simulink model "dt_crff3_non_ideal"  (R2025b)
settings: Solver=VariableStepAuto  StartTime=0.0  StopTime=10.0  RelTol=1e-3
model workspace (MAT data in the model file):
  Delay_1 = [0 0 0]
  ENOB_1 = 3.82010676042
  FUNDF_1 = [99.7346662356 299.517854363]
  FUNDX_1 = [15.4853229373 -15.5048641556]
  IMODF_1 = [nan 499.461934629]
  IMODX_1 = [nan -22.9176650349]
  NoiseFloor_1 = -39.8464180971
  OIP3_1 = nan
  SFDR_1 = 30.038334306
  SINAD_1 = 24.7570426978
  SNR_1 = 26.1601373132
  THD_1 = -30.1916968059
  delay_1 = [0 0 0]
undefined symbols (not defined in the file): DiscIntNeverNeededParam, Fs
libraries: dspmlti4 x5, msbAdcMeasurements x1, cstblocks x1, dspobslib x1, simulink x1
settings Model: Creator=divya  LastModifiedBy=divya

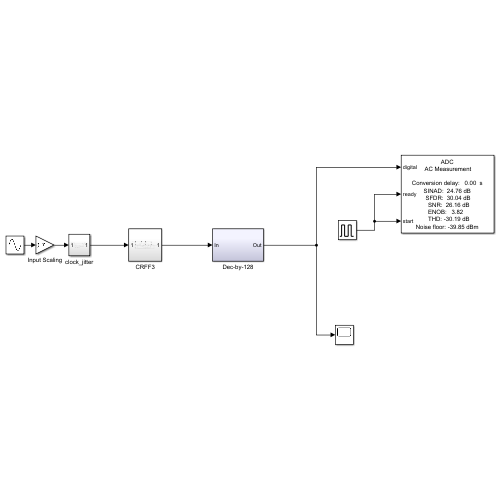
[thumbnail: Simulink's stored preview of the top-level diagram]
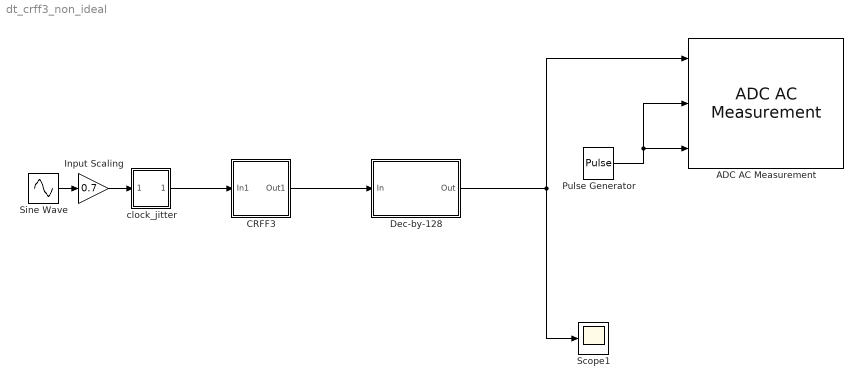
== system dt_crff3_non_ideal ==
  ADC AC Measurement : msbAdcMeasurements/ADC AC Measurement  DistortionMeasurement=Harmonic  InputFrequency=100  Method=Filter bank (slower, requires extra simulation time)  RBW=0.97656  AutoSetRBW=on  NBits=18  Frequency=512e3/512  HoldOffTime=0  OutputToWorkspace=on  VariableName=adc_ac_out  ShowSpectrum=off
      link override ADC AC Measurement/ADC AC Measurement Spectrum Analyzer: YLimits=[-137.7231 -38.3847]
  CRFF3 : Subsystem
  Dec-by-128 : Subsystem  Tag=BlockMethodSubSystem
  Input Scaling : Gain  Gain=0.7
  Pulse Generator : DiscretePulseGenerator  PulseType=Time based  Period=1/1e3  PulseWidth=50
  Scope1 : Scope
      settings: ActiveDisplayYMinimum=-0.48077534934995808  ActiveDisplayYMaximum=0.47749694685441174
  Sine Wave : Sin  Amplitude=0.5  Frequency=628  SampleTime=0
  clock_jitter : Subsystem
  wires:
  Sine Wave/1 -> Input Scaling/1
  clock_jitter/1(Out1) -> CRFF3/1(In1)
  Input Scaling/1 -> clock_jitter/1(In1)
  Pulse Generator/1 -> ADC AC Measurement/3, ADC AC Measurement/2
  Dec-by-128/1(Out) -> ADC AC Measurement/1, Scope1/1
  CRFF3/1(Out1) -> Dec-by-128/1(In)

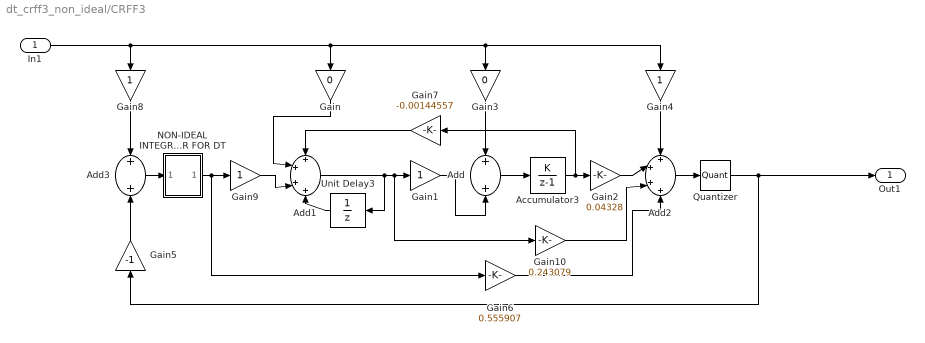
== system dt_crff3_non_ideal/CRFF3 ==
  In1 : Inport
  Accumulator3 : DiscreteIntegrator  RequirementInfo={} %GIDa_84b8a85e_70bd_4012_ac1e_63614c4be6d6  IntegratorMethod=Accumulation: Forward Euler  SampleTime=1/(2e3*256)  ICPrevOutput=DiscIntNeverNeededParam  ICPrevScaledInput=DiscIntNeverNeededParam
  Add : Sum  RequirementInfo={} %GIDa_1bae6441_7ec0_4b3d_934d_76e9e43c9b7e
  Add1 : Sum  RequirementInfo={} %GIDa_a9ab647b_ef6c_44ae_a7d7_07674ff6e1b7  Inputs=++++
  Add2 : Sum  RequirementInfo={} %GIDa_90ab26b4_1233_497e_bd04_95e33db7a632  Inputs=++++
  Add3 : Sum  RequirementInfo={} %GIDa_7332c942_930d_40b4_92c2_cb866450a1ff
  Gain : Gain  RequirementInfo={} %GIDa_66f1e292_dda5_4196_a756_d7da6c9f4ec1  Gain=0
  Gain1 : Gain  RequirementInfo={} %GIDa_65ba529b_3bb8_47a6_991c_193e84d935ec
  Gain10 : Gain  RequirementInfo={} %GIDa_9d9f86ed_3f68_4820_a7bb_2b036d160bea  Gain=0.243079
  Gain2 : Gain  RequirementInfo={} %GIDa_aff9fc4e_08da_4d4c_a30b_0e4ade6494bf  Gain=0.04328
  Gain3 : Gain  RequirementInfo={} %GIDa_9119ba48_5aaa_4b92_8d55_fe7266434502  Gain=0
  Gain4 : Gain  RequirementInfo={} %GIDa_0e2722ef_9053_4d44_905a_33326b2b6931
  Gain5 : Gain  RequirementInfo={} %GIDa_f0a11f36_a50f_4b52_8fee_37920b06259d  Gain=-1
  Gain6 : Gain  RequirementInfo={} %GIDa_c76b328f_db54_4ce8_9437_510e711bab7a  Gain=0.555907
  Gain7 : Gain  RequirementInfo={} %GIDa_74793299_c4f9_4dc2_b47d_1811f6d964e4  Gain=-0.00144557
  Gain8 : Gain  RequirementInfo={} %GIDa_eaa10ee5_6284_4d1e_87e1_14929015d833
  Gain9 : Gain  RequirementInfo={} %GIDa_87574565_9502_45cc_a9fb_7b5e642d0bb9
  NON-IDEAL INTEGRATOR FOR DT : Subsystem
  Quantizer : Quantizer  RequirementInfo={} %GIDa_8abe0c8b_02fb_4844_986b_6a962a179ce5  QuantizationInterval=1
  Unit Delay3 : UnitDelay  SampleTime=1/(2e3*256)  HasFrameUpgradeWarning=on
  Out1 : Outport
  wires:
  Gain6/1 -> Add2/4
  Add1/1 -> Unit Delay3/1, Gain10/1, Gain1/1
  Accumulator3/1 -> Gain7/1, Gain2/1
  NON-IDEAL INTEGRATOR FOR DT/1(Out1) -> Gain9/1, Gain6/1
  Unit Delay3/1 -> Add1/4
  Gain9/1 -> Add1/3
  Gain8/1 -> Add3/1
  In1/1 -> Gain8/1, Gain/1, Gain3/1, Gain4/1
  Gain5/1 -> Add3/2
  Gain2/1 -> Add2/2
  Gain10/1 -> Add2/3
  Gain3/1 -> Add/1
  Gain/1 -> Add1/2
  Add2/1 -> Quantizer/1
  Gain7/1 -> Add1/1
  Quantizer/1 -> Out1/1, Gain5/1
  Gain4/1 -> Add2/1
  Gain1/1 -> Add/2
  Add3/1 -> NON-IDEAL INTEGRATOR FOR DT/1(In2)
  Add/1 -> Accumulator3/1

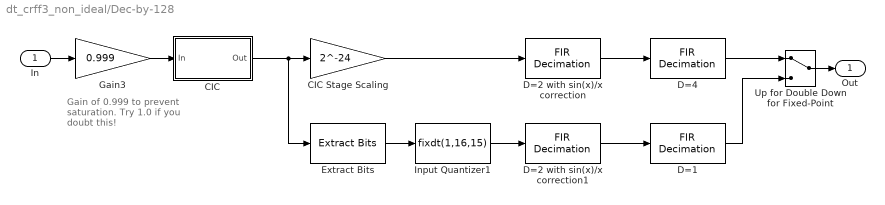
== system dt_crff3_non_ideal/Dec-by-128 ==
  note: Gain of 0.999
      |  to prevent saturation.
      | Try 1.0 if you doubt this!
  In : Inport
  CIC : Subsystem  Tag=BlockMethodSubSystem
  CIC Stage Scaling : Gain  Gain=2^-24  OutDataTypeStr=double
  D=1 : dspmlti4/FIR Decimation  Tag=BlockMethodSubSystem  FilterSource=Dialog parameters  h=[3.91622882568566e-005 6.87965858042108e-005 -4.54214374064863e-005 -0.000494371495641253 -0.00130180300923401 -0.00208967903904167 -0.00212227242054207 -0.000820466891279789 0.00150204580522739 0.00336930831020411 0.00293785704853453 -0.000377156856911545 -0.00470730589029979 -0.00641725180832836 -0.00285434238807273 0.00468881704747952 0.0106481610663031 0.00886595641260817 -0.00177682957707149 -0.0144760924096176 -0.0180887636371107 -0.00603326390232397 0.0159987454589339 0.0309930177585429 0.0221515825094605 -0.011846123967549 -0.04979943488328 -0.0572170491759349 -0.00847489358036981 0.0923226139783473 0.207458472082029 0.283964644704709 0.283964644704709 0.207458472082029 0.0923226139783473 -0.00847489358036981 -0.0572170491759349 -0.04979943488328 -0.011846123967549 0.0221515825094605 0.0309930177585429 0.0159987454589339 -0.00603326390232397 -0.0180887636371107 -0.0144760924096176 -0.00177682957707149 0.00886595641260817 0.0106481610663031 0.00468881704747952 -0.00285434238807273 -0.00641725180832836 -0.00470730589029979 -0.000377156856911545 0.00293785704853453 0.00336930831020411 0.00150204580522739 -0.000820466891279789 -0.00212227242054207 -0.00208967903904167 -0.00130180300923401 -0.000494371495641253 -4.54214374064863e-005 6.87965858042108e-005 3.91622882568566e-005]  D=4  filtStruct=Direct form  FilterObject=Hm_firdecim  framing=Allow multirate processing  AllowArbitraryInputLength=off  inputOffset=0  outputBufInitCond=0  roundingMode=Floor  overflowMode=off  firstCoeffMode=Binary point scaling  firstCoeffWordLength=16  firstCoeffFracLength=16  firstCoeffDataTypeStr=fixdt(1,16,16)  firstCoeffMin=[]  firstCoeffMax=[]  firstCoeffLastDataTypeStr=fixdt(1,16,16)  outputMin=[]  outputMax=[]
  D=2 with sin(x)/x correction : dspmlti4/FIR Decimation  Tag=BlockMethodSubSystem  FilterSource=Dialog parameters  h=[0.000549322570782159 0.0028188201427819 0.00605408312993028 0.00388745313496409 -0.0121134249050654 -0.0371670852364025 -0.0412525748188521 0.0145135665847005 0.134839839295902 0.264505645586551 0.320972309879795 0.264505645586551 0.134839839295902 0.0145135665847005 -0.0412525748188521 -0.0371670852364025 -0.0121134249050654 0.00388745313496409 0.00605408312993028 0.0028188201427819 0.000549322570782159]  D=2  filtStruct=Direct form  FilterObject=Hm_firdecim  framing=Allow multirate processing  AllowArbitraryInputLength=off  inputOffset=0  outputBufInitCond=0  roundingMode=Floor  overflowMode=off  firstCoeffDataTypeStr=Inherit: Same word length as input  firstCoeffMin=[]  firstCoeffMax=[]  firstCoeffLastDataTypeStr=Inherit: Same word length as input  outputDataTypeStr=Inherit: Same as accumulator  outputMin=[]  outputMax=[]  outputLastDataTypeStr=Inherit: Same as accumulator
  D=2 with sin(x)/x correction1 : dspmlti4/FIR Decimation  Tag=BlockMethodSubSystem  FilterSource=Dialog parameters  h=[0.000549322570782159 0.0028188201427819 0.00605408312993028 0.00388745313496409 -0.0121134249050654 -0.0371670852364025 -0.0412525748188521 0.0145135665847005 0.134839839295902 0.264505645586551 0.320972309879795 0.264505645586551 0.134839839295902 0.0145135665847005 -0.0412525748188521 -0.0371670852364025 -0.0121134249050654 0.00388745313496409 0.00605408312993028 0.0028188201427819 0.000549322570782159]  D=2  filtStruct=Direct form  FilterObject=Hm_firdecim  framing=Allow multirate processing  AllowArbitraryInputLength=off  inputOffset=0  outputBufInitCond=0  roundingMode=Floor  overflowMode=off  firstCoeffMode=Binary point scaling  firstCoeffWordLength=16  firstCoeffFracLength=16  firstCoeffDataTypeStr=fixdt(1,16,16)  firstCoeffMin=[]  firstCoeffMax=[]  firstCoeffLastDataTypeStr=fixdt(1,16,16)  outputMin=[]  outputMax=[]
  D=4 : dspmlti4/FIR Decimation  Tag=BlockMethodSubSystem  FilterSource=Dialog parameters  h=[3.91622882568566e-005 6.87965858042108e-005 -4.54214374064863e-005 -0.000494371495641253 -0.00130180300923401 -0.00208967903904167 -0.00212227242054207 -0.000820466891279789 0.00150204580522739 0.00336930831020411 0.00293785704853453 -0.000377156856911545 -0.00470730589029979 -0.00641725180832836 -0.00285434238807273 0.00468881704747952 0.0106481610663031 0.00886595641260817 -0.00177682957707149 -0.0144760924096176 -0.0180887636371107 -0.00603326390232397 0.0159987454589339 0.0309930177585429 0.0221515825094605 -0.011846123967549 -0.04979943488328 -0.0572170491759349 -0.00847489358036981 0.0923226139783473 0.207458472082029 0.283964644704709 0.283964644704709 0.207458472082029 0.0923226139783473 -0.00847489358036981 -0.0572170491759349 -0.04979943488328 -0.011846123967549 0.0221515825094605 0.0309930177585429 0.0159987454589339 -0.00603326390232397 -0.0180887636371107 -0.0144760924096176 -0.00177682957707149 0.00886595641260817 0.0106481610663031 0.00468881704747952 -0.00285434238807273 -0.00641725180832836 -0.00470730589029979 -0.000377156856911545 0.00293785704853453 0.00336930831020411 0.00150204580522739 -0.000820466891279789 -0.00212227242054207 -0.00208967903904167 -0.00130180300923401 -0.000494371495641253 -4.54214374064863e-005 6.87965858042108e-005 3.91622882568566e-005]  D=4  filtStruct=Direct form  FilterObject=Hm_firdecim  framing=Allow multirate processing  AllowArbitraryInputLength=off  inputOffset=0  outputBufInitCond=0  roundingMode=Floor  overflowMode=off  firstCoeffDataTypeStr=Inherit: Same word length as input  firstCoeffMin=[]  firstCoeffMax=[]  firstCoeffLastDataTypeStr=Inherit: Same word length as input  outputDataTypeStr=Inherit: Same as accumulator  outputMin=[]  outputMax=[]  outputLastDataTypeStr=Inherit: Same as accumulator
  Extract Bits : simulink/Logic and Bit Operations/Extract Bits  bitsToExtract=Upper half  numBits=8  bitIdxRange=[0 7]  outScalingMode=Treat bit field as an integer
  Gain3 : Gain  Gain=0.999
  Input Quantizer1 : DataTypeConversion  OutDataTypeStr=fixdt(1,16,15)  ConvertRealWorld=Stored Integer (SI)  RndMeth=Round
  Up for Double Down for Fixed-Point : ManualSwitch
  Out : Outport  VectorParamsAs1DForOutWhenUnconnected=off
  wires:
  In/1 -> Gain3/1
  CIC/1(Out) -> CIC Stage Scaling/1, Extract Bits/1
  CIC Stage Scaling/1 -> D=2 with sin(x)/x correction/1
  Gain3/1 -> CIC/1(In)
  Input Quantizer1/1 -> D=2 with sin(x)/x correction1/1
  Extract Bits/1 -> Input Quantizer1/1
  D=2 with sin(x)/x correction1/1 -> D=1/1
  D=4/1 -> Up for Double Down for Fixed-Point/1
  D=1/1 -> Up for Double Down for Fixed-Point/2
  Up for Double Down for Fixed-Point/1 -> Out/1
  D=2 with sin(x)/x correction/1 -> D=4/1

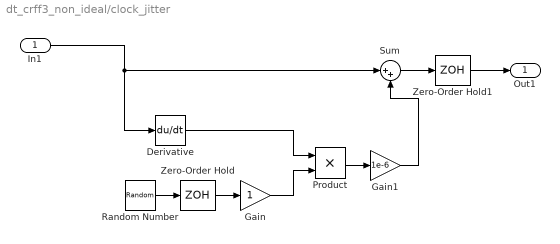
== system dt_crff3_non_ideal/clock_jitter ==
  In1 : Inport
  Derivative : Derivative
  Gain : Gain
  Gain1 : Gain  Gain=1e-6
  Product : Product
  Random Number : RandomNumber  SampleTime=0.1
  Sum : Sum  Inputs=|++
  Zero-Order Hold : ZeroOrderHold  SampleTime=-1
  Zero-Order Hold1 : ZeroOrderHold  SampleTime=1/512e3
  Out1 : Outport
  wires:
  In1/1 -> Derivative/1, Sum/1
  Derivative/1 -> Product/1
  Zero-Order Hold1/1 -> Out1/1
  Sum/1 -> Zero-Order Hold1/1
  Random Number/1 -> Zero-Order Hold/1
  Zero-Order Hold/1 -> Gain/1
  Gain/1 -> Product/2
  Product/1 -> Gain1/1
  Gain1/1 -> Sum/2

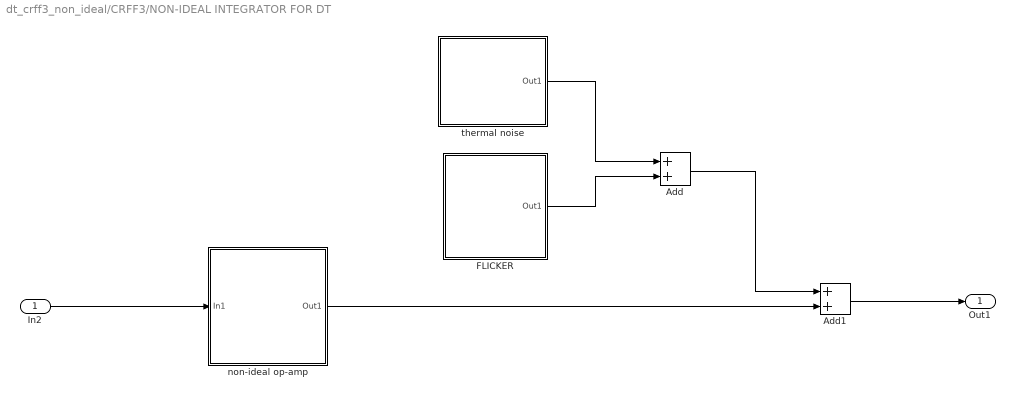
== system dt_crff3_non_ideal/CRFF3/NON-IDEAL INTEGRATOR FOR DT ==
  In2 : Inport
  Add : Sum
  Add1 : Sum
  FLICKER : Subsystem
  "non-ideal op-amp " : Subsystem
  thermal noise : Subsystem
  Out1 : Outport
  wires:
  In2/1 -> "non-ideal op-amp "/1(In1)
  Add/1 -> Add1/1
  Add1/1 -> Out1/1
  "non-ideal op-amp "/1(Out1) -> Add1/2
  thermal noise/1(Out1) -> Add/1
  FLICKER/1(Out1) -> Add/2

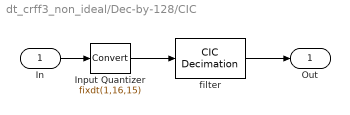
== system dt_crff3_non_ideal/Dec-by-128/CIC ==
  In : Inport
  Input Quantizer : DataTypeConversion  OutDataTypeStr=fixdt(1,16,15)  RndMeth=Round
  filter : dspmlti4/CIC Decimation  filtFrom=Dialog parameters  filtobj=Hm_decim  ftype=Decimator  R=64  M=1  N=4  filterInternals=Full precision  BPS=[32 32 32 32 32 32 32 32]  FLPS=[15 15 15 15 15 15 15 15]  outputWordLength=32  outputFracLength=15  launchFVT=off  framing=Maintain input frame rate  RateOptions=Allow multirate processing
  Out : Outport  VectorParamsAs1DForOutWhenUnconnected=off
  wires:
  In/1 -> Input Quantizer/1
  Input Quantizer/1 -> filter/1
  filter/1 -> Out/1

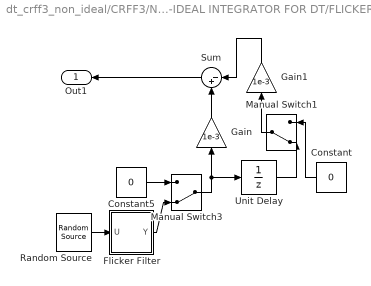
== system dt_crff3_non_ideal/CRFF3/NON-IDEAL INTEGRATOR FOR DT/FLICKER ==
  Constant : Constant  Value=0
  Constant5 : Constant  Value=0  SampleTime=1/Fs
  Flicker Filter : Subsystem
  Gain : Gain  Gain=1e-3
  Gain1 : Gain  Gain=1e-3
  Manual Switch1 : ManualSwitch  CurrentSetting=0
  Manual Switch3 : ManualSwitch  CurrentSetting=0
  Random Source : dspobslib/Random Source  SrcType=Gaussian  NormMethod=Ziggurat  CltLength=12  MinVal=0  MaxVal=1  MeanVal=0  VarVal=1  RepMode=Not repeatable  rawSeed=1  IsInherit=off  SampMode=Discrete  SampTime=1/Fs  SampFrame=1  DataType=Double  OutComplex=Real  OutputFrames=off
  Sum : Sum  Inputs=|-+
  Unit Delay : UnitDelay  SampleTime=1/Fs  HasFrameUpgradeWarning=on
  Out1 : Outport
  wires:
  Manual Switch3/1 -> Gain/1, Unit Delay/1
  Random Source/1 -> Flicker Filter/1(U)
  Unit Delay/1 -> Manual Switch1/2
  Constant5/1 -> Manual Switch3/1
  Constant/1 -> Manual Switch1/1
  Gain/1 -> Sum/2
  Flicker Filter/1(Y) -> Manual Switch3/2
  Sum/1 -> Out1/1
  Manual Switch1/1 -> Gain1/1
  Gain1/1 -> Sum/1

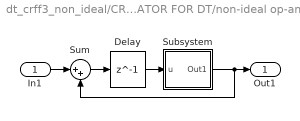
== system dt_crff3_non_ideal/CRFF3/NON-IDEAL INTEGRATOR FOR DT/non-ideal op-amp  ==
  In1 : Inport
  Delay : Delay  DelayLength=1  InputProcessing=Columns as channels (frame based)  SampleTime=1/(2e3*128)
  Subsystem : Subsystem
  Sum : Sum  Inputs=|++
  Out1 : Outport
  wires:
  Subsystem/1(Out1) -> Out1/1, Sum/2
  In1/1 -> Sum/1
  Sum/1 -> Delay/1
  Delay/1 -> Subsystem/1(u)

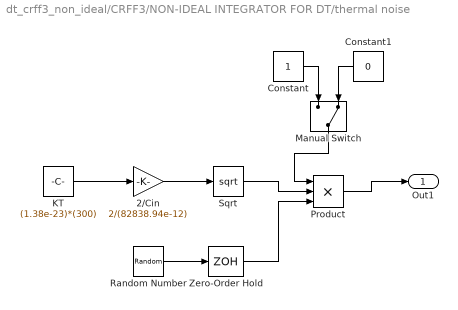
== system dt_crff3_non_ideal/CRFF3/NON-IDEAL INTEGRATOR FOR DT/thermal noise ==
  2/Cin : Gain  Gain=2/(82838.94e-12)
  Constant : Constant
  Constant1 : Constant  Value=0
  KT : Constant  Value=(1.38e-23)*(300)
  Manual Switch : ManualSwitch  CurrentSetting=0
  Product : Product  Inputs=3
  Random Number : RandomNumber  SampleTime=0.1
  Sqrt : Sqrt
  Zero-Order Hold : ZeroOrderHold  SampleTime=1/(2e3*128)
  Out1 : Outport
  wires:
  Product/1 -> Out1/1
  Random Number/1 -> Zero-Order Hold/1
  KT/1 -> 2/Cin/1
  2/Cin/1 -> Sqrt/1
  Constant1/1 -> Manual Switch/2
  Constant/1 -> Manual Switch/1
  Zero-Order Hold/1 -> Product/3
  Sqrt/1 -> Product/2
  Manual Switch/1 -> Product/1

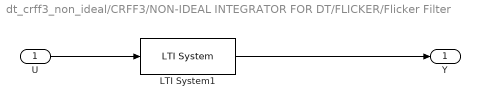
== system dt_crff3_non_ideal/CRFF3/NON-IDEAL INTEGRATOR FOR DT/FLICKER/Flicker Filter ==
  U : Inport
  LTI System1 : cstblocks/LTI System  sys=ff_dt  IC=[]  PadeOrder=0
  Y : Outport
  wires:
  LTI System1/1 -> Y/1
  U/1 -> LTI System1/1

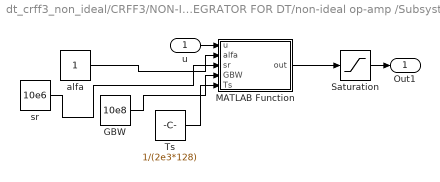
== system dt_crff3_non_ideal/CRFF3/NON-IDEAL INTEGRATOR FOR DT/non-ideal op-amp /Subsystem ==
  u : Inport
  GBW : Constant  Value=10e8
  MATLAB Function : MATLAB Function  TreatAsAtomicUnit=on
  Saturation : Saturate  UpperLimit=0.7  LowerLimit=-0.7
  Ts : Constant  Value=1/(2e3*128)
  alfa : Constant
  sr : Constant  Value=10e6
  Out1 : Outport
  wires:
  Ts/1 -> MATLAB Function/5(Ts)
  MATLAB Function/1(out) -> Saturation/1
  alfa/1 -> MATLAB Function/2(alfa)
  GBW/1 -> MATLAB Function/4(GBW)
  sr/1 -> MATLAB Function/3(sr)
  Saturation/1 -> Out1/1
  u/1 -> MATLAB Function/1(u)

== matlab function dt_crff3_non_ideal/CRFF3/NON-IDEAL INTEGRATOR FOR DT/non-ideal op-amp /Subsystem/MATLAB Function ==
  data: u input; out output; alfa input; sr input; GBW input; Ts input
function out = slew(u, alfa, sr, GBW, Ts)
% Models the op-amp slew rate for a discrete-time integrator
% u    : input signal amplitude (Vp - Vn)
% alfa : finite gain effect (A0/(1+A0)), ideal op-amp alfa = 1
% sr   : slew rate in V/s
% GBW  : gain-bandwidth of op-amp (Hz)
% Ts   : sample time (s)

tau = 1/(2*pi*GBW);   % time constant
Tmax = Ts/2;           % discrete half-step
slope = alfa * abs(u) / tau;

if slope > sr
    % Op-amp is slewing
    tsl = abs(u)*alfa/sr - tau;   % slewing time
    
    if tsl >= Tmax
        % fully slewing entire half period
        error = abs(u) - sr*Tmax;
    else
        % partial slewing, partial linear region
        texp = Tmax - tsl;
        error = abs(u)*(1-alfa) + (alfa*abs(u) - sr*tsl) * exp(-texp/tau);
    end
    
else
    % Linear region (no slewing)
    texp = Tmax;
    error = abs(u)*(1-alfa) + alfa*abs(u)*exp(-texp/tau);
end

out = u - sign(u)*error;
